simulink model "solenoid"  (Simulink 7.0)
settings: Solver=ode45  StartTime=0.0  StopTime=0.03  RelTol=1e-3
settings Model: Creator=binaryblade  LastModifiedBy=binaryblade
settings DataIOCC: LimitDataPoints=off
settings DebuggingCC: AlgebraicLoopMsg=none

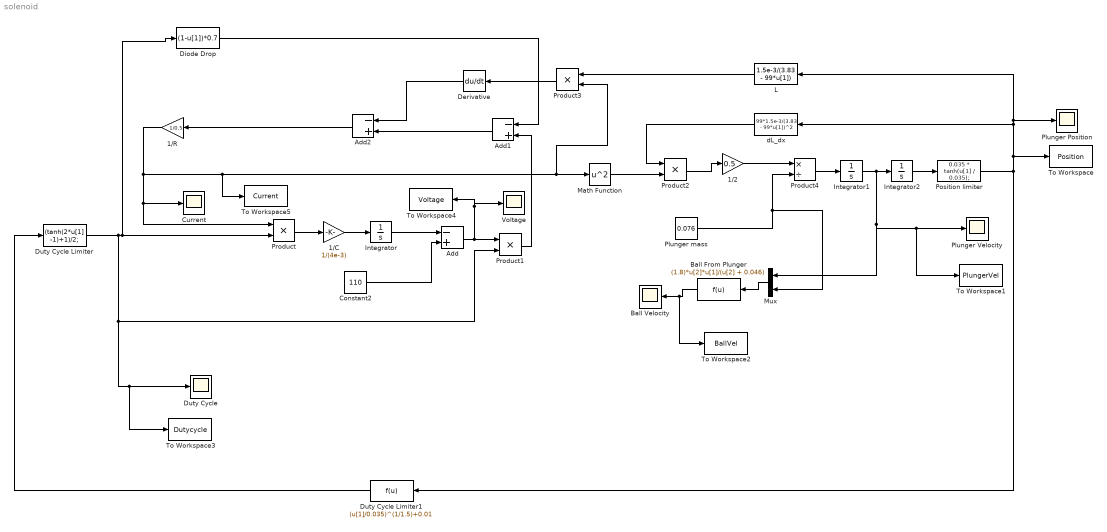
== system solenoid ==
  1/2 : Gain  Gain=0.5  ParameterDataType=sfix(16)  ParameterScaling=2^0  OutDataType=sfix(16)  OutScaling=2^0
  1/C : Gain  Gain=1/(4e-3)  ParameterDataType=sfix(16)  ParameterScaling=2^0  OutDataType=sfix(16)  OutScaling=2^0
  1/R : Gain  Orientation=left  Gain=1/0.5  ParameterDataType=sfix(16)  ParameterScaling=2^0  OutDataType=sfix(16)  OutScaling=2^0
  Add : Sum  Inputs=-+  OutDataType=sfix(16)  OutScaling=2^-10
  Add1 : Sum  Orientation=left  Inputs=-+  OutDataType=sfix(16)  OutScaling=2^-10
  Add2 : Sum  Orientation=left  Inputs=-+  OutDataType=sfix(16)  OutScaling=2^-10
  Ball From Plunger : Fcn  Orientation=left  Expr=(1.8)*u[2]*u[1]/(u[2] + 0.046)
  Ball Velocity : Scope
      settings: SaveName=ScopeData3
  Constant2 : Constant  Value=110  OutDataType=sfix(16)  OutScaling=2^0
  Current : Scope
  Derivative : Derivative  Orientation=left
  Diode Drop : Fcn  Expr=(1-u[1])*0.7
  Duty Cycle : Scope
      settings: SaveName=ScopeData5
  Duty Cycle Limiter : Fcn  Expr=(tanh(2*u[1] -1)+1)/2;
  Duty Cycle Limiter1 : Fcn  Orientation=left  Expr=(u[1]/0.035)^(1/1.5)+0.01
  Integrator : Integrator
  Integrator1 : Integrator
  Integrator2 : Integrator
  L : Fcn  Orientation=left  Expr=1.5e-3/(3.83 - 99*u[1])
  Math Function : Math  Operator=square  OutDataType=sfix(16)  OutScaling=2^0  SaturateOnIntegerOverflow=on
  Mux : Mux  Orientation=left  Inputs=2
  Plunger Position : Scope
  Plunger Velocity : Scope
      settings: SaveName=ScopeData2
  Plunger mass : Constant  Value=0.076  OutDataType=sfix(16)  OutScaling=2^0
  Position limiter : Fcn  Expr="0.035 * tanh(u[1]  / 0.035);"
  Product : Product  OutDataType=sfix(16)  OutScaling=2^0  RndMeth=Zero
  Product1 : Product  OutDataType=sfix(16)  OutScaling=2^0  RndMeth=Zero
  Product2 : Product  OutDataType=sfix(16)  OutScaling=2^0  RndMeth=Zero
  Product3 : Product  Orientation=left  OutDataType=sfix(16)  OutScaling=2^0  RndMeth=Zero
  Product4 : Product  Inputs=*/  OutDataType=sfix(16)  OutScaling=2^0  RndMeth=Zero
  To Workspace : ToWorkspace  VariableName=Position  SampleTime=-1  SaveFormat=Array
  To Workspace1 : ToWorkspace  VariableName=PlungerVel  SampleTime=-1  SaveFormat=Array
  To Workspace2 : ToWorkspace  VariableName=BallVel  SampleTime=-1  SaveFormat=Array
  To Workspace3 : ToWorkspace  VariableName=Dutycycle  SampleTime=-1  SaveFormat=Array
  To Workspace4 : ToWorkspace  VariableName=Voltage  SampleTime=-1  SaveFormat=Array
  To Workspace5 : ToWorkspace  VariableName=Current  SampleTime=-1  SaveFormat=Array
  Voltage : Scope
      settings: SaveName=ScopeData4
  dL_dx : Fcn  Orientation=left  Expr=99*1.5e-3/(3.83 - 99*u[1])^2
  wires:
  Product/1 -> 1/C/1
  1/C/1 -> Integrator/1
  Integrator/1 -> Add/1
  Constant2/1 -> Add/2
  Add/1 -> Product1/1, Voltage/1, To Workspace4/1
  Product1/1 -> Add1/2
  Diode Drop/1 -> Add1/1
  Add1/1 -> Add2/2
  Add2/1 -> 1/R/1
  1/R/1 -> Product/1, Current/1, Math Function/1, Product3/2, To Workspace5/1
  Derivative/1 -> Add2/1
  Math Function/1 -> Product2/2
  Product2/1 -> 1/2/1
  1/2/1 -> Product4/1
  Integrator1/1 -> Integrator2/1, Mux/1, Plunger Velocity/1, To Workspace1/1
  Product3/1 -> Derivative/1
  L/1 -> Product3/1
  dL_dx/1 -> Product2/1
  Plunger mass/1 -> Product4/2, Mux/2
  Ball From Plunger/1 -> Ball Velocity/1, To Workspace2/1
  Mux/1 -> Ball From Plunger/1
  Product4/1 -> Integrator1/1
  Integrator2/1 -> Position limiter/1
  Position limiter/1 -> Plunger Position/1, L/1, dL_dx/1, To Workspace/1, Duty Cycle Limiter1/1
  Duty Cycle Limiter/1 -> Product/2, Diode Drop/1, Product1/2, Duty Cycle/1, To Workspace3/1
  Duty Cycle Limiter1/1 -> Duty Cycle Limiter/1
